simulink model "simulation"  (R2016b)
settings: Solver=ode4  StartTime=0.0  StopTime=15  FixedStep=1e-4  MaxStep=0.01  RelTol=1e-4  EnableMultiTasking=on
libraries: cstblocks x2
settings Model: Creator=furieril  LastModifiedBy=furieril
settings DataIOCC: LimitDataPoints=on  SaveOutput=off  SaveTime=off
settings OptimizationCC: ExpressionDepthLimit=2147483647  LifeSpan=1
settings DebuggingCC: UnderspecifiedInitializationDetection=Classic  MergeDetectMultiDrivingBlocksExec=none  FcnCallInpInsideContextMsg=warning  AllowSymbolicDim=off  StateNameClashWarn=warning  SFUnexpectedBacktrackingDiag=warning  SFNoUnconditionalDefaultTransitionDiag=warning  SFExecutionAtInitializationDiag=none
settings GRTTargetCC: TargetLangStandard=C89/C90 (ANSI)  GeneratePreprocessorConditionals=Disable all  CombineOutputUpdateFcns=off  GRTInterface=on

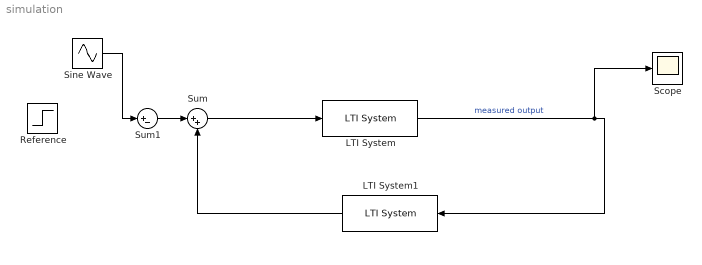
== system simulation ==
  LTI System : cstblocks/LTI System  sys=Gmodel  IC=[]
  LTI System1 : cstblocks/LTI System  sys=Kmodel2  IC=[]
  Reference : Step  SampleTime=0
  Scope : Scope
  Sine Wave : Sin  Frequency=100  SampleTime=0
  Sum : Sum  Inputs=|++
  Sum1 : Sum  Inputs=|+-
  wires:
  LTI System/1 -> Scope/1, LTI System1/1  "measured output"
  Sum/1 -> LTI System/1
  Sum1/1 -> Sum/1
  Sine Wave/1 -> Sum1/1
  LTI System1/1 -> Sum/2
